simulink model "manualControl"  (R2017a)
settings: Solver=FixedStepDiscrete  StartTime=0.0  StopTime=Inf  FixedStep=0.1  RelTol=1e-3  EnableMultiTasking=on
model workspace (MAT data in the model file):
  SL_ROS_VariableLengthArrays_MaxSizes.CommonInfo.ArrayTruncateAction = 'EmitWarning'
  SL_ROS_VariableLengthArrays_MaxSizes.MsgTypeMap = containers.Map
  SL_ROS_VariableLengthArrays_MaxSizes.MsgTypeMap.serialization.keys = {'sensor_msgs/Image', 'sensor_msgs/LaserScan'}
  SL_ROS_VariableLengthArrays_MaxSizes.MsgTypeMap.serialization.values{1}(1).PropertyName = 'Data'
  SL_ROS_VariableLengthArrays_MaxSizes.MsgTypeMap.serialization.values{1}(1).DataType = 'uint8'
  SL_ROS_VariableLengthArrays_MaxSizes.MsgTypeMap.serialization.values{1}(1).MaxLength = 691200
  SL_ROS_VariableLengthArrays_MaxSizes.MsgTypeMap.serialization.values{1}(2).PropertyName = 'Encoding'
  SL_ROS_VariableLengthArrays_MaxSizes.MsgTypeMap.serialization.values{1}(2).DataType = 'uint8'
  SL_ROS_VariableLengthArrays_MaxSizes.MsgTypeMap.serialization.values{1}(2).MaxLength = 128
  SL_ROS_VariableLengthArrays_MaxSizes.MsgTypeMap.serialization.values{2}(1).PropertyName = 'Intensities'
  SL_ROS_VariableLengthArrays_MaxSizes.MsgTypeMap.serialization.values{2}(1).DataType = 'single'
  SL_ROS_VariableLengthArrays_MaxSizes.MsgTypeMap.serialization.values{2}(1).MaxLength = 1081
  SL_ROS_VariableLengthArrays_MaxSizes.MsgTypeMap.serialization.values{2}(2).PropertyName = 'Ranges'
  SL_ROS_VariableLengthArrays_MaxSizes.MsgTypeMap.serialization.values{2}(2).DataType = 'single'
  SL_ROS_VariableLengthArrays_MaxSizes.MsgTypeMap.serialization.values{2}(2).MaxLength = 1081
  SL_ROS_VariableLengthArrays_MaxSizes.MsgTypeMap.serialization.uniformity = 0
  SL_ROS_VariableLengthArrays_MaxSizes.MsgTypeMap.serialization.keyType = 'char'
  SL_ROS_VariableLengthArrays_MaxSizes.MsgTypeMap.serialization.valueType = 'any'
undefined symbols (not defined in the file): Angular, gray, Linear
libraries: robotlib x6, aerolibanimutils x1, simulink x1
settings Model: Creator=The MathWorks, Inc.  LastModifiedBy=jcassett
settings DataIOCC: LimitDataPoints=on  SaveFormat=Array
settings OptimizationCC: LifeSpan=Inf  MaxStackSize=64
settings DebuggingCC: SolverPrmCheckMsg=warning  SFUnexpectedBacktrackingDiag=warning  SFNoUnconditionalDefaultTransitionDiag=warning  SFExecutionAtInitializationDiag=none
settings HardwareCC: ProdBitPerPointer=32  ProdBitPerSizeT=32  ProdBitPerPtrDiffT=32  ProdLargestAtomicFloat=None  ProdIntDivRoundTo=Undefined  ProdEndianess=Unspecified  ProdWordSize=32  ProdHWDeviceType=Generic->Unspecified (assume 32-bit Generic)  UseEmbeddedCoderFeatures=off
settings ModelReferenceCC: PropagateSignalLabelsOutOfModel=off
settings RTWCC: SystemTargetFile=ert.tlc  HardwareBoard=Robot Operating System (ROS)  TLCOptions=-aInlineSetEventsForThisBaseRateFcn=TLC_FALSE -aSuppressMultiTaskScheduler=TLC_FALSE -aRateBasedStepFcn=0  TemplateMakefile=ert_default_tmf  Description=Embedded Coder  Toolchain=Catkin  TargetLang=C++
settings ERTTargetCC: MultiwordLength=2048  ERTCustomFileBanners=off  SupportContinuousTime=on  SupportNonInlinedSFcns=on  RemoveResetFunc=off  SupportVariableSizeSignals=on  ModelStepFunctionPrototypeControlCompliant=off  ConvertIfToSwitch=off  SuppressUnreachableDefaultCases=off
settings ConfigComp: CovMetricSettings=dw  CovHtmlReporting=on  CovSaveCumulativeToWorkspaceVar=on  CovSaveSingleToWorkspaceVar=on  CovExternalEMLEnable=off  CovSFcnEnable=off

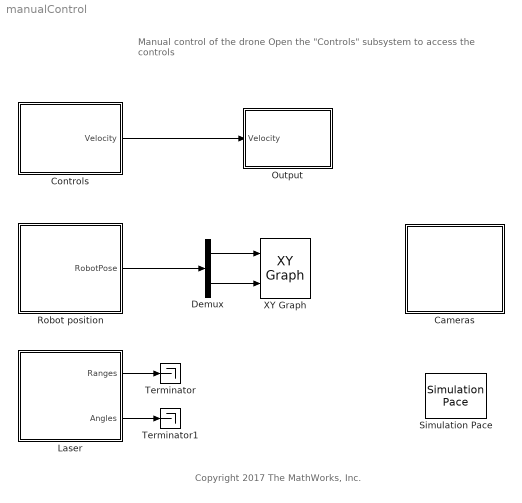
== system manualControl ==
  note: Manual control of the drone
      | Open the "Controls" subsystem to access the controls
  note: Copyright 2017 The MathWorks, Inc.
  Cameras : Subsystem
  Controls : Subsystem
  Demux : Demux  Outputs=2
  Laser : Subsystem
  Output : Subsystem
  Robot position : Subsystem
  Simulation Pace : aerolibanimutils/Simulation Pace  SimulationPace=1  SleepMode=MATLAB Thread  OutputPaceError=off  SampleTime=-1
  Terminator : Terminator
  Terminator1 : Terminator
  XY Graph : simulink/Sinks/XY Graph  xmin=-10  xmax=30  ymin=-10  ymax=10  st=-1
  wires:
  Controls/1(Velocity) -> Output/1(Velocity)
  Robot position/1(RobotPose) -> Demux/1
  Demux/1 -> XY Graph/1
  Demux/2 -> XY Graph/2
  Laser/1(Ranges) -> Terminator/1
  Laser/2(Angles) -> Terminator1/1

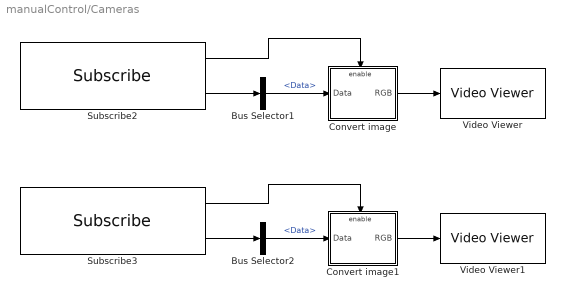
== system manualControl/Cameras ==
  Bus Selector1 : BusSelector  DialogController=Simulink.DDGSource_BusSelector  OutputSignals=Data
  Bus Selector2 : BusSelector  DialogController=Simulink.DDGSource_BusSelector  OutputSignals=Data
  Convert image : Subsystem
  Convert image1 : Subsystem
  Subscribe2 : robotlib/Subscribe  SourceLibraryInfo=This block requires Robotics System Toolbox  topicSource=Select from ROS network  topic=/quadrotor_1/front/image_raw  messageType=sensor_msgs/Image  sampleTime=-1  messageQueueLength=51
      settings: SourceProductBaseCode=RO
  Subscribe3 : robotlib/Subscribe  SourceLibraryInfo=This block requires Robotics System Toolbox  topicSource=Select from ROS network  topic=/quadrotor_1/bottom/image_raw  messageType=sensor_msgs/Image  sampleTime=-1  messageQueueLength=51
      settings: SourceProductBaseCode=RO
  Video Viewer : VideoViewer  colormapValue=gray(256)  FigPos=[1022.09090909091 508.545454545455 609.163636363637 376.145454545455]
  Video Viewer1 : VideoViewer  colormapValue=gray(256)  FigPos=[1013.36363636364 1003.38181818182 609.163636363636 376.145454545455]
  wires:
  Subscribe2/1 -> Convert image/Enable
  Convert image1/1(RGB) -> Video Viewer1/1
  Subscribe3/2 -> Bus Selector2/1
  Subscribe2/2 -> Bus Selector1/1
  Bus Selector1/1 -> Convert image/1(Data)  "<Data>"
  Bus Selector2/1 -> Convert image1/1(Data)  "<Data>"
  Subscribe3/1 -> Convert image1/Enable
  Convert image/1(RGB) -> Video Viewer/1

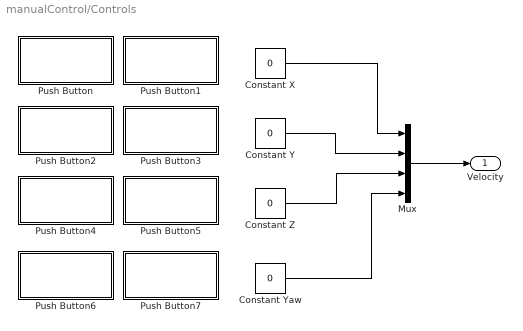
== system manualControl/Controls ==
  Constant X : Constant  Value=0
  Constant Y : Constant  Value=0
  Constant Yaw : Constant  Value=0
  Constant Z : Constant  Value=0
  Mux : Mux
  Push Button : Subsystem  DialogController=hmiCreateDDGDialog  IsWebBlock=on  mask(MWDashboardBlock){webBlockId=8823c1c9-d070-41d1-8454-48132908df2a, webBlockType=pushbutton, ShowInLibBrwoser=on, ShowInitialText=on, HMISrcModelName=manualControl}
      mask prompts: webBlockId "WebBlock Id"; webBlockType "WebBlock Type"; HMISrcModelName "Source Model"
      mask help: SimulinkHMI:dialogs:PushButtonDialogDesc
      mask Help: helpview([docroot '/mapfiles/simulink.map'], 'hmi_push_button')
      mask Display:
      | model = bdroot(gcb);
      | if strcmp(get_param(model,'BlockDiagramType'), 'library')
      |     image([(matlabroot) '/toolbox/simulink/hmi/icons/PushButton.png']);
      | end
  Push Button1 : Subsystem  DialogController=hmiCreateDDGDialog  IsWebBlock=on  mask(MWDashboardBlock){webBlockId=565e639a-c5b4-412c-83c7-fee4de231406, webBlockType=pushbutton, ShowInLibBrwoser=on, ShowInitialText=on, HMISrcModelName=manualControl}
      mask prompts: webBlockId "WebBlock Id"; webBlockType "WebBlock Type"; HMISrcModelName "Source Model"
      mask help: SimulinkHMI:dialogs:PushButtonDialogDesc
      mask Help: helpview([docroot '/mapfiles/simulink.map'], 'hmi_push_button')
      mask Display:
      | model = bdroot(gcb);
      | if strcmp(get_param(model,'BlockDiagramType'), 'library')
      |     image([(matlabroot) '/toolbox/simulink/hmi/icons/PushButton.png']);
      | end
  Push Button2 : Subsystem  DialogController=hmiCreateDDGDialog  IsWebBlock=on  mask(MWDashboardBlock){webBlockId=11d88ad8-289e-4346-bb92-ac02d79fbabe, webBlockType=pushbutton, ShowInLibBrwoser=on, ShowInitialText=on, HMISrcModelName=manualControl}
      mask prompts: webBlockId "WebBlock Id"; webBlockType "WebBlock Type"; HMISrcModelName "Source Model"
      mask help: SimulinkHMI:dialogs:PushButtonDialogDesc
      mask Help: helpview([docroot '/mapfiles/simulink.map'], 'hmi_push_button')
      mask Display:
      | model = bdroot(gcb);
      | if strcmp(get_param(model,'BlockDiagramType'), 'library')
      |     image([(matlabroot) '/toolbox/simulink/hmi/icons/PushButton.png']);
      | end
  Push Button3 : Subsystem  DialogController=hmiCreateDDGDialog  IsWebBlock=on  mask(MWDashboardBlock){webBlockId=aaf97ce7-b473-428d-bb9d-b9ec47914714, webBlockType=pushbutton, ShowInLibBrwoser=on, ShowInitialText=on, HMISrcModelName=manualControl}
      mask prompts: webBlockId "WebBlock Id"; webBlockType "WebBlock Type"; HMISrcModelName "Source Model"
      mask help: SimulinkHMI:dialogs:PushButtonDialogDesc
      mask Help: helpview([docroot '/mapfiles/simulink.map'], 'hmi_push_button')
      mask Display:
      | model = bdroot(gcb);
      | if strcmp(get_param(model,'BlockDiagramType'), 'library')
      |     image([(matlabroot) '/toolbox/simulink/hmi/icons/PushButton.png']);
      | end
  Push Button4 : Subsystem  DialogController=hmiCreateDDGDialog  IsWebBlock=on  mask(MWDashboardBlock){webBlockId=6121c4fa-0a5d-4952-9203-d734a374474b, webBlockType=pushbutton, ShowInLibBrwoser=on, ShowInitialText=on, HMISrcModelName=manualControl}
      mask prompts: webBlockId "WebBlock Id"; webBlockType "WebBlock Type"; HMISrcModelName "Source Model"
      mask help: SimulinkHMI:dialogs:PushButtonDialogDesc
      mask Help: helpview([docroot '/mapfiles/simulink.map'], 'hmi_push_button')
      mask Display:
      | model = bdroot(gcb);
      | if strcmp(get_param(model,'BlockDiagramType'), 'library')
      |     image([(matlabroot) '/toolbox/simulink/hmi/icons/PushButton.png']);
      | end
  Push Button5 : Subsystem  DialogController=hmiCreateDDGDialog  IsWebBlock=on  mask(MWDashboardBlock){webBlockId=aec6c2e6-6bd1-4372-8d02-c5a459e73747, webBlockType=pushbutton, ShowInLibBrwoser=on, ShowInitialText=on, HMISrcModelName=manualControl}
      mask prompts: webBlockId "WebBlock Id"; webBlockType "WebBlock Type"; HMISrcModelName "Source Model"
      mask help: SimulinkHMI:dialogs:PushButtonDialogDesc
      mask Help: helpview([docroot '/mapfiles/simulink.map'], 'hmi_push_button')
      mask Display:
      | model = bdroot(gcb);
      | if strcmp(get_param(model,'BlockDiagramType'), 'library')
      |     image([(matlabroot) '/toolbox/simulink/hmi/icons/PushButton.png']);
      | end
  Push Button6 : Subsystem  DialogController=hmiCreateDDGDialog  IsWebBlock=on  mask(MWDashboardBlock){webBlockId=b9a66a52-21de-4d85-9b8e-2dbbcceec934, webBlockType=pushbutton, ShowInLibBrwoser=on, ShowInitialText=on, HMISrcModelName=manualControl}
      mask prompts: webBlockId "WebBlock Id"; webBlockType "WebBlock Type"; HMISrcModelName "Source Model"
      mask help: SimulinkHMI:dialogs:PushButtonDialogDesc
      mask Help: helpview([docroot '/mapfiles/simulink.map'], 'hmi_push_button')
      mask Display:
      | model = bdroot(gcb);
      | if strcmp(get_param(model,'BlockDiagramType'), 'library')
      |     image([(matlabroot) '/toolbox/simulink/hmi/icons/PushButton.png']);
      | end
  Push Button7 : Subsystem  DialogController=hmiCreateDDGDialog  IsWebBlock=on  mask(MWDashboardBlock){webBlockId=d1f340f7-9c41-4830-b0c6-21d6a447c6d4, webBlockType=pushbutton, ShowInLibBrwoser=on, ShowInitialText=on, HMISrcModelName=manualControl}
      mask prompts: webBlockId "WebBlock Id"; webBlockType "WebBlock Type"; HMISrcModelName "Source Model"
      mask help: SimulinkHMI:dialogs:PushButtonDialogDesc
      mask Help: helpview([docroot '/mapfiles/simulink.map'], 'hmi_push_button')
      mask Display:
      | model = bdroot(gcb);
      | if strcmp(get_param(model,'BlockDiagramType'), 'library')
      |     image([(matlabroot) '/toolbox/simulink/hmi/icons/PushButton.png']);
      | end
  Velocity : Outport
  wires:
  Mux/1 -> Velocity/1
  Constant Y/1 -> Mux/2
  Constant X/1 -> Mux/1
  Constant Z/1 -> Mux/3
  Constant Yaw/1 -> Mux/4

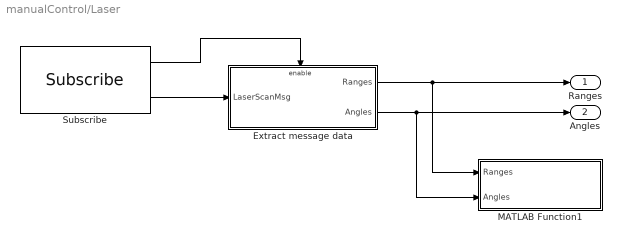
== system manualControl/Laser ==
  Extract message data : Subsystem
  MATLAB Function1 : MATLAB Function  TreatAsAtomicUnit=on
  Subscribe : robotlib/Subscribe  SourceLibraryInfo=This block requires Robotics System Toolbox  topicSource=Select from ROS network  topic=/quadrotor_1/scan  messageType=sensor_msgs/LaserScan  sampleTime=-1  messageQueueLength=1
      settings: SourceProductBaseCode=RO
  Ranges : Outport
  Angles : Outport  Port=2
  wires:
  Subscribe/1 -> Extract message data/Enable
  Extract message data/2(Angles) -> Angles/1, MATLAB Function1/2(Angles)
  Subscribe/2 -> Extract message data/1(LaserScanMsg)
  Extract message data/1(Ranges) -> Ranges/1, MATLAB Function1/1(Ranges)

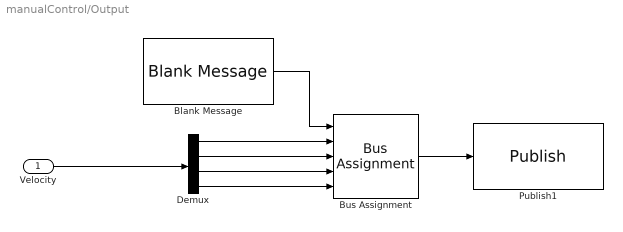
== system manualControl/Output ==
  Velocity : Inport
  Blank Message : robotlib/Blank Message  SourceLibraryInfo=This block requires Robotics System Toolbox  messageType=geometry_msgs/Twist  SampleTime=0
      settings: SourceProductBaseCode=RO
  Bus Assignment : BusAssignment  DialogController=Simulink.DDGSource_BusAssignment  AssignedSignals=Linear.X,Linear.Y,Linear.Z,Angular.Z
  Demux : Demux
  Publish1 : robotlib/Publish  SourceLibraryInfo=This block requires Robotics System Toolbox  topicSource=Select from ROS network  topic=/quadrotor_1/cmd_vel  messageType=geometry_msgs/Twist  messageQueueLength=105
      settings: SourceProductBaseCode=RO
  wires:
  Demux/2 -> Bus Assignment/3
  Demux/1 -> Bus Assignment/2
  Demux/3 -> Bus Assignment/4
  Demux/4 -> Bus Assignment/5
  Velocity/1 -> Demux/1
  Bus Assignment/1 -> Publish1/1
  Blank Message/1 -> Bus Assignment/1

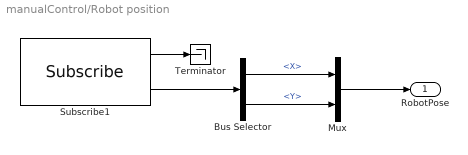
== system manualControl/Robot position ==
  Bus Selector : BusSelector  DialogController=Simulink.DDGSource_BusSelector  OutputSignals=Pose.Pose.Position.X,Pose.Pose.Position.Y
  Mux : Mux  Inputs=2
  Subscribe1 : robotlib/Subscribe  SourceLibraryInfo=This block requires Robotics System Toolbox  topicSource=Select from ROS network  topic=/quadrotor_1/ground_truth/state  messageType=nav_msgs/Odometry  sampleTime=-1  messageQueueLength=51
      settings: SourceProductBaseCode=RO
  Terminator : Terminator
  RobotPose : Outport
  wires:
  Subscribe1/2 -> Bus Selector/1
  Subscribe1/1 -> Terminator/1
  Bus Selector/1 -> Mux/1  "<X>"
  Bus Selector/2 -> Mux/2  "<Y>"
  Mux/1 -> RobotPose/1

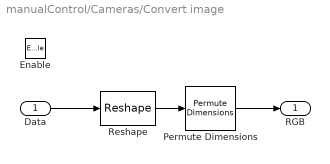
== system manualControl/Cameras/Convert image ==
  Data : Inport
  Enable : EnablePort
  Permute Dimensions : PermuteDimensions  Order=[3 2 1]
  Reshape : Reshape  OutputDimensionality=Customize  OutputDimensions=[3 640 360]
  RGB : Outport
  wires:
  Permute Dimensions/1 -> RGB/1
  Reshape/1 -> Permute Dimensions/1
  Data/1 -> Reshape/1

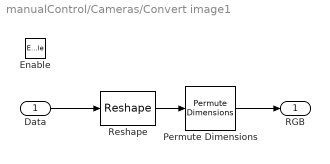
== system manualControl/Cameras/Convert image1 ==
  Data : Inport
  Enable : EnablePort
  Permute Dimensions : PermuteDimensions  Order=[3 2 1]
  Reshape : Reshape  OutputDimensionality=Customize  OutputDimensions=[3 640 360]
  RGB : Outport
  wires:
  Permute Dimensions/1 -> RGB/1
  Reshape/1 -> Permute Dimensions/1
  Data/1 -> Reshape/1

== system manualControl/Controls/Push Button ==

== system manualControl/Controls/Push Button1 ==

== system manualControl/Controls/Push Button2 ==

== system manualControl/Controls/Push Button3 ==

== system manualControl/Controls/Push Button4 ==

== system manualControl/Controls/Push Button5 ==

== system manualControl/Controls/Push Button6 ==

== system manualControl/Controls/Push Button7 ==

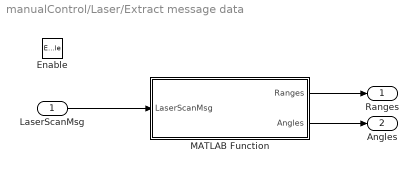
== system manualControl/Laser/Extract message data ==
  LaserScanMsg : Inport
  Enable : EnablePort
  MATLAB Function : MATLAB Function  TreatAsAtomicUnit=on
  Ranges : Outport
  Angles : Outport  Port=2
  wires:
  MATLAB Function/1(Ranges) -> Ranges/1
  MATLAB Function/2(Angles) -> Angles/1
  LaserScanMsg/1 -> MATLAB Function/1(LaserScanMsg)

== matlab function manualControl/Laser/MATLAB Function1 ==
  data: Ranges input; Angles input
function plotLaser(Ranges, Angles)
coder.extrinsic('polarplot');
persistent p;
if isempty(p)
    p = polarplot(0, 0, '.');
    set(gca, 'ThetaZeroLocation', 'top', 'ThetaLim', [-135 135], ...
        'RAxisLocation', 0, 'RLim', [0 10]);
end
if ishandle(p)
    set(p, 'ThetaData', Angles);
    set(p, 'RData', Ranges);
    drawnow limitrate;
end

== matlab function manualControl/Laser/Extract message data/MATLAB Function ==
  data: LaserScanMsg input; Ranges output size=[1081 1]; Angles output size=[1081 1]
function [Ranges, Angles] = ExtractRangeData(LaserScanMsg)
%#codegen

% Extract Range information
Ranges = double(LaserScanMsg.Ranges);

% Construct Angles vector using AngleMin and AngleIncrement from sensor
% reading.
angMin = double(LaserScanMsg.AngleMin);
angMax = double(LaserScanMsg.AngleMax);
rawAngles = linspace(angMax, angMin, numel(Ranges)).';

% Wrap the angles to the (-pi,pi] interval.
Angles = robotics.internal.wrapToPi(double(rawAngles));
